simulink model "ratc_sim"  (R2016a)
settings: Solver=FixedStepAuto  StartTime=0.0  StopTime=100  RelTol=1e-3
undefined symbols (not defined in the file or in its folder): P, U_trim, X_trim
libraries: X8_lib x2, simulink x1
settings Model: Creator=andreanv  LastModifiedBy=andreanv

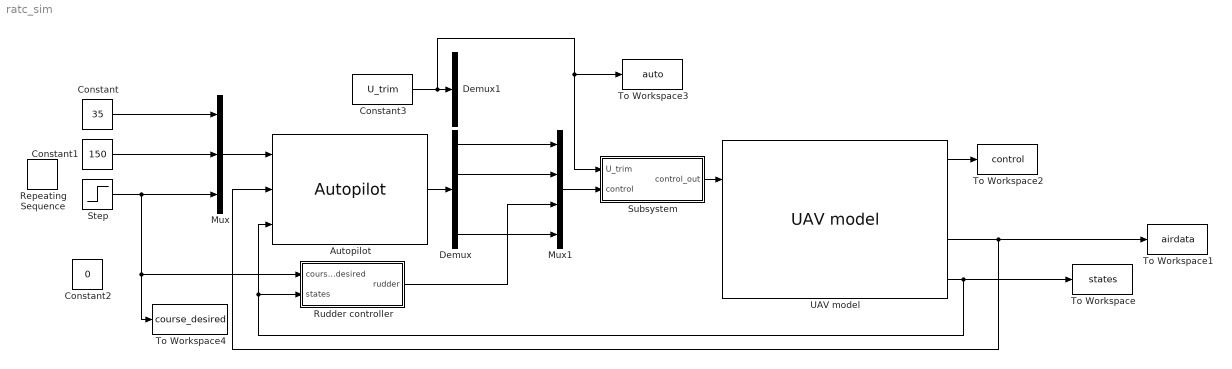
== system ratc_sim ==
  Autopilot : X8_lib/Autopilot  param=param  X_trim=X_trim  U_trim=[-0.0594 0.0005 -0.0010 0.0978]'
  Constant : Constant  Value=35
  Constant1 : Constant  Value=150
  Constant2 : Constant  Value=0
  Constant3 : Constant  Value=U_trim
  Demux : Demux
  Demux1 : Demux
  Mux : Mux  Inputs=3
  Mux1 : Mux
  Repeating Sequence : simulink/Sources/Repeating Sequence  rep_seq_t=[0 100]  rep_seq_y=[0 0]
  Rudder controller : Subsystem
  Step : Step  Time=50  After=pi/4  SampleTime=0
  Subsystem : Subsystem
  To Workspace : ToWorkspace  VariableName=states  SaveFormat=Timeseries  SampleTime=-1
  To Workspace1 : ToWorkspace  VariableName=airdata  SaveFormat=Timeseries  SampleTime=-1
  To Workspace2 : ToWorkspace  VariableName=control  SaveFormat=Timeseries  SampleTime=-1
  To Workspace3 : ToWorkspace  VariableName=auto  SaveFormat=Timeseries  SampleTime=-1
  To Workspace4 : ToWorkspace  VariableName=course_desired  SaveFormat=Timeseries  SampleTime=-1
  UAV model : X8_lib/UAV model  param=param  pos0=X_trim(1:3)'  quat0=X_trim(4:7)'  vel0=X_trim(8:10)'  rate0=X_trim(11:13)'  servoR_pos0=X_trim(14)  servoR_vel0=X_trim(15)  servoL_pos0=X_trim(16)  servoL_vel0=X_trim(17)  motor_speed0=X_trim(18)
  wires:
  UAV model/4 -> Autopilot/3, Rudder controller/2(states), To Workspace/1
  UAV model/3 -> Autopilot/2, To Workspace1/1
  Mux/1 -> Autopilot/1
  Constant/1 -> Mux/1
  Constant1/1 -> Mux/2
  UAV model/1 -> To Workspace2/1
  Constant3/1 -> Subsystem/1(U_trim), To Workspace3/1, Demux1/1
  Autopilot/1 -> Demux/1
  Demux/2 -> Mux1/2
  Subsystem/1(control_out) -> UAV model/1
  Mux1/1 -> Subsystem/2(control)
  Demux/1 -> Mux1/1
  Demux/4 -> Mux1/4
  Rudder controller/1(rudder) -> Mux1/3
  Step/1 -> Rudder controller/1(course_desired), To Workspace4/1, Mux/3

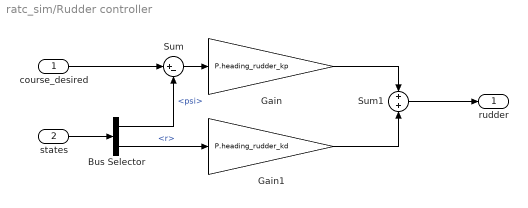
== system ratc_sim/Rudder controller ==
  course_desired : Inport
  states : Inport  Port=2
  Bus Selector : BusSelector  OutputSignals=Attitude.psi,AngularVelocity.r
  Gain : Gain  Gain=P.heading_rudder_kp
  Gain1 : Gain  Gain=P.heading_rudder_kd
  Sum : Sum  Inputs=|+-
  Sum1 : Sum  Inputs=+|+
  rudder : Outport
  wires:
  states/1 -> Bus Selector/1
  course_desired/1 -> Sum/1
  Bus Selector/1 -> Sum/2  "<psi>"
  Sum/1 -> Gain/1
  Bus Selector/2 -> Gain1/1  "<r>"
  Gain1/1 -> Sum1/2
  Gain/1 -> Sum1/1
  Sum1/1 -> rudder/1

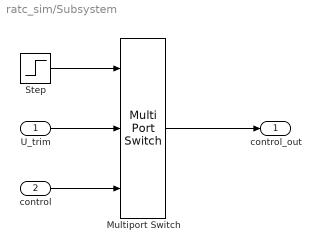
== system ratc_sim/Subsystem ==
  U_trim : Inport
  control : Inport  Port=2
  Multiport Switch : MultiPortSwitch  Inputs=2
  Step : Step  Time=2  Before=1  After=2  SampleTime=0
  control_out : Outport
  wires:
  U_trim/1 -> Multiport Switch/2
  control/1 -> Multiport Switch/3
  Multiport Switch/1 -> control_out/1
  Step/1 -> Multiport Switch/1
